simulink model "CMOS_Kernel_Memory_Sync"  (R2023b)
settings: Solver=VariableStepAuto  StartTime=0.0  StopTime=30000000  RelTol=1e-3
values from neighbouring files (symbols this model uses):
  AmountOfPixelsPerScanline = 400    [Kernel_Setup_Script.m]
  AmountOfRamBlocksScanlines = 5    [Kernel_Setup_Script.m]
  AmountOfRamBlocksScanlinesOffset = AmountOfRamBlocksScanlines - 1    (= 4)    [Kernel_Setup_Script.m]
  AmountOfScanlinePixels = 73700    [Kernel_Setup_Script.m]
  AmountOfScanlinePixelsOffset = AmountOfScanlinePixels - 1    (= 73699)    [Kernel_Setup_Script.m]
  AmountOfScanlines = 1100    [Kernel_Setup_Script.m]
  AmountOfScanlinesOffset = AmountOfScanlines - 1    (= 1099)    [Kernel_Setup_Script.m]
  AOPPK_Off = AmountOfPixelsPerScanline - 1    (= 399)    [Kernel_Setup_Script.m]
  AOPPS_Off = AmountOfPixelsPerScanline - 1    (= 399)    [Kernel_Setup_Script.m]
  FramePackOff_0 = FramePackOff_0 - ScanlineFifoCheck    [Kernel_Setup_Script.m]
  FramePackOff_1 = FramePackOff_1 - ScanlineFifoCheck    [Kernel_Setup_Script.m]
  FramePackOff_2 = FramePackOff_2 - ScanlineFifoCheck    [Kernel_Setup_Script.m]
  FramePackOff_3 = FramePackOff_3 - ScanlineFifoCheck    [Kernel_Setup_Script.m]
  FramePackOff_4 = FramePackOff_4 - ScanlineFifoCheck    [Kernel_Setup_Script.m]
  FramePackOff_5 = FramePackOff_5 - ScanlineFifoCheck    [Kernel_Setup_Script.m]
  KernelPackOff_0 = KernelPackOff_0 - KernelBitsPerRow    [Kernel_Setup_Script.m]
  KernelPackOff_1 = KernelPackOff_1 - KernelBitsPerRow    [Kernel_Setup_Script.m]
  KernelPackOff_2 = KernelPackOff_2 - KernelBitsPerRow    [Kernel_Setup_Script.m]
  KernelPackOff_3 = KernelPackOff_3 - KernelBitsPerRow    [Kernel_Setup_Script.m]
  Slice59DownTo48Top = (MsbOffset - (ScanlinePixelBitSizeController*1))    (= 59)    [Kernel_Setup_Script.m]
  Slice71DownTo60Top = (MsbOffset - (ScanlinePixelBitSizeController*0))    (= 71)    [Kernel_Setup_Script.m]
  TotalSectionsForFrames = AmountOfScanlines/AmountOfRamBlocksScanlines    (= 220)    [Kernel_Setup_Script.m]
  UltraRamRows = AmountOfPixelsPerScanline/ScanlineFifoCheck    [Kernel_Setup_Script.m]
  UltraRamRowsCeil = ceil(AmountOfPixelsPerScanline/ScanlineFifoCheck)    [Kernel_Setup_Script.m]
  UltraRamRowsKernel = AmountOfPixelsPerScanline/KernelBitsPerRow    (= 100)    [Kernel_Setup_Script.m]
  UltraRamRowsKernelCeil = ceil(AmountOfPixelsPerScanline/KernelBitsPerRow)    [Kernel_Setup_Script.m]
  UltraRamRowsMemorySectionOffset = UltraRamRowsCeil*AmountOfRamBlocksScanlines    [Kernel_Setup_Script.m]
  UltraRamRowsOffset = UltraRamRowsCeil - 1    [Kernel_Setup_Script.m]
undefined symbols (not defined in the file or in its folder): c, Down, sfvc784, Up, xck26
libraries: hdlBasic x4512, vmcUtilities x1
(part 4 of 39)

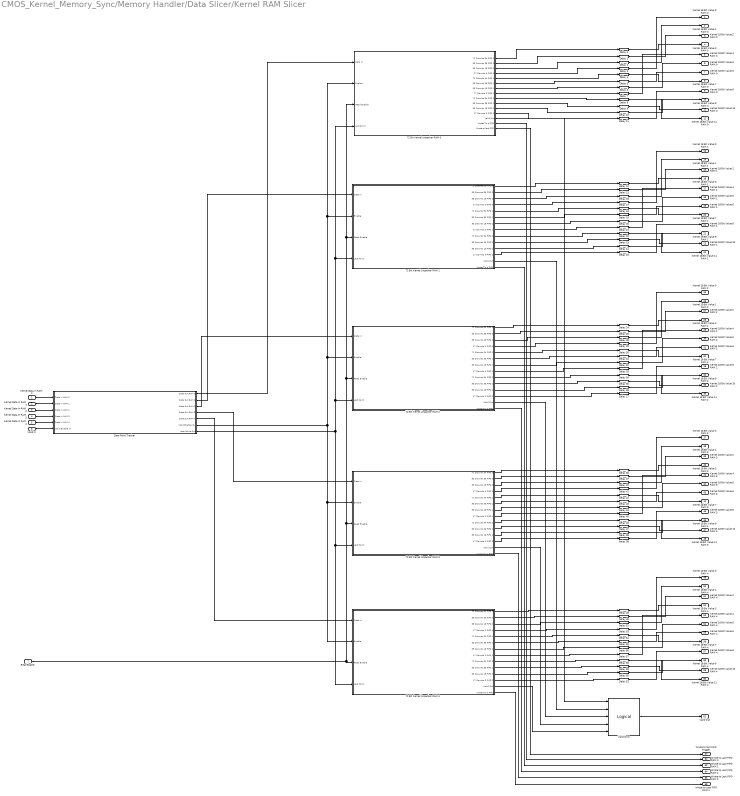
== system CMOS_Kernel_Memory_Sync/Memory Handler/Data Slicer/Kernel RAM Slicer ==
  Kernel Data In RAM 0 : Inport
  Kernel Data In RAM 1 : Inport  Port=2
  Kernel Data In RAM 2 : Inport  Port=3
  Kernel Data In RAM 3 : Inport  Port=4
  Kernel Data In RAM 4 : Inport  Port=5
  Valid In : Inport  Port=6
  Read Enable : Inport  Port=7
  72 Bit Kernel Unpacker RAM 0 : Subsystem
      settings: RTWMemSecFuncInitTerm=Inherit fRAM model  RTWMemSecFuncExecute=Inherit fRAM model  RTWMemSecDataConstants=Inherit fRAM model  RTWMemSecDataInternal=Inherit fRAM model  RTWMemSecDataParameters=Inherit fRAM model
  72 Bit Kernel Unpacker RAM 1 : Subsystem
      settings: RTWMemSecFuncInitTerm=Inherit fRAM model  RTWMemSecFuncExecute=Inherit fRAM model  RTWMemSecDataConstants=Inherit fRAM model  RTWMemSecDataInternal=Inherit fRAM model  RTWMemSecDataParameters=Inherit fRAM model
  72 Bit Kernel Unpacker RAM 2 : Subsystem
      settings: RTWMemSecFuncInitTerm=Inherit fRAM model  RTWMemSecFuncExecute=Inherit fRAM model  RTWMemSecDataConstants=Inherit fRAM model  RTWMemSecDataInternal=Inherit fRAM model  RTWMemSecDataParameters=Inherit fRAM model
  72 Bit Kernel Unpacker RAM 3 : Subsystem
      settings: RTWMemSecFuncInitTerm=Inherit fRAM model  RTWMemSecFuncExecute=Inherit fRAM model  RTWMemSecDataConstants=Inherit fRAM model  RTWMemSecDataInternal=Inherit fRAM model  RTWMemSecDataParameters=Inherit fRAM model
  72 Bit Kernel Unpacker RAM 4 : Subsystem
      settings: RTWMemSecFuncInitTerm=Inherit fRAM model  RTWMemSecFuncExecute=Inherit fRAM model  RTWMemSecDataConstants=Inherit fRAM model  RTWMemSecDataInternal=Inherit fRAM model  RTWMemSecDataParameters=Inherit fRAM model
  Data Point Tracker : Subsystem
  Delay {0..59} (60 alike) : hdlBasic/Delay  rst=off  en=off  latency=1  reg_retiming=off  XmcBlockStatus=1  maskContainerNames=group1  block_type=delay  block_config=sysgen:Delay_config
  Valid Sync : hdlBasic/Logical  logical_function=AND  inputs=5  en=off  latency=1  precision=Full  arith_type=Unsigned  n_bits=16  bin_pt=0  align_bp=on  overflow=[]  quantization=[]  XmcBlockStatus=1  maskContainerNames=tabcontainer1  block_type=logical  block_config=sysgen:Logical_config
  Kernel 18 Bit Value 0 RAM 0 : Outport
  Kernel 18 Bit Value 1 RAM 0 : Outport  Port=2
  Kernel 18 Bit Value 2 RAM 0 : Outport  Port=3
  Kernel 18 Bit Value 3 RAM 0 : Outport  Port=4
  Kernel 18 Bit Value 4 RAM 0 : Outport  Port=5
  Kernel 18 Bit Value 5 RAM 0 : Outport  Port=6
  Kernel 18 Bit Value 6 RAM 0 : Outport  Port=7
  Kernel 18 Bit Value 7 RAM 0 : Outport  Port=8
  Kernel 18 Bit Value 8 RAM 0 : Outport  Port=9
  Kernel 18 Bit Value 9 RAM 0 : Outport  Port=10
  Kernel 18 Bit Value 10 RAM 0 : Outport  Port=11
  Kernel 18 Bit Value 11 RAM 0 : Outport  Port=12
  Kernel 18 Bit Value 0 RAM 1 : Outport  Port=13
  Kernel 18 Bit Value 1 RAM 1 : Outport  Port=14
  Kernel 18 Bit Value 2 RAM 1 : Outport  Port=15
  Kernel 18 Bit Value 3 RAM 1 : Outport  Port=16
  Kernel 18 Bit Value 4 RAM 1 : Outport  Port=17
  Kernel 18 Bit Value 5 RAM 1 : Outport  Port=18
  Kernel 18 Bit Value 6 RAM 1 : Outport  Port=19
  Kernel 18 Bit Value 7 RAM 1 : Outport  Port=20
  Kernel 18 Bit Value 8 RAM 1 : Outport  Port=21
  Kernel 18 Bit Value 9 RAM 1 : Outport  Port=22
  Kernel 18 Bit Value 10 RAM 1 : Outport  Port=23
  Kernel 18 Bit Value 11 RAM 1 : Outport  Port=24
  Kernel 18 Bit Value 0 RAM 2 : Outport  Port=25
  Kernel 18 Bit Value 1 RAM 2 : Outport  Port=26
  Kernel 18 Bit Value 2 RAM 2 : Outport  Port=27
  Kernel 18 Bit Value 3 RAM 2 : Outport  Port=28
  Kernel 18 Bit Value 4 RAM 2 : Outport  Port=29
  Kernel 18 Bit Value 5 RAM 2 : Outport  Port=30
  Kernel 18 Bit Value 6 RAM 2 : Outport  Port=31
  Kernel 18 Bit Value 7 RAM 2 : Outport  Port=32
  Kernel 18 Bit Value 8 RAM 2 : Outport  Port=33
  Kernel 18 Bit Value 9 RAM 2 : Outport  Port=34
  Kernel 18 Bit Value 10 RAM 2 : Outport  Port=35
  Kernel 18 Bit Value 11 RAM 2 : Outport  Port=36
  Kernel 18 Bit Value 0 RAM 3 : Outport  Port=37
  Kernel 18 Bit Value 1 RAM 3 : Outport  Port=38
  Kernel 18 Bit Value 2 RAM 3 : Outport  Port=39
  Kernel 18 Bit Value 3 RAM 3 : Outport  Port=40
  Kernel 18 Bit Value 4 RAM 3 : Outport  Port=41
  Kernel 18 Bit Value 5 RAM 3 : Outport  Port=42
  Kernel 18 Bit Value 6 RAM 3 : Outport  Port=43
  Kernel 18 Bit Value 7 RAM 3 : Outport  Port=44
  Kernel 18 Bit Value 8 RAM 3 : Outport  Port=45
  Kernel 18 Bit Value 9 RAM 3 : Outport  Port=46
  Kernel 18 Bit Value 10 RAM 3 : Outport  Port=47
  Kernel 18 Bit Value 11 RAM 3 : Outport  Port=48
  Kernel 18 Bit Value 0 RAM 4 : Outport  Port=49
  Kernel 18 Bit Value 1 RAM 4 : Outport  Port=50
  Kernel 18 Bit Value 2 RAM 4 : Outport  Port=51
  Kernel 18 Bit Value 3 RAM 4 : Outport  Port=52
  Kernel 18 Bit Value 4 RAM 4 : Outport  Port=53
  Kernel 18 Bit Value 5 RAM 4 : Outport  Port=54
  Kernel 18 Bit Value 6 RAM 4 : Outport  Port=55
  Kernel 18 Bit Value 7 RAM 4 : Outport  Port=56
  Kernel 18 Bit Value 8 RAM 4 : Outport  Port=57
  Kernel 18 Bit Value 9 RAM 4 : Outport  Port=58
  Kernel 18 Bit Value 10 RAM 4 : Outport  Port=59
  Kernel 18 Bit Value 11 RAM 4 : Outport  Port=60
  Valid Out : Outport  Port=61
  Wrote to Last FIFO RAM 0 : Outport  Port=62
  Wrote to Last FIFO RAM 1 : Outport  Port=63
  Wrote to Last FIFO RAM 2 : Outport  Port=64
  Wrote to Last FIFO RAM 3 : Outport  Port=65
  Wrote to Last FIFO RAM 4 : Outport  Port=66
  Wrote to last FIFO Trigger : Outport  Port=67
  wires:
  72 Bit Kernel Unpacker RAM 0/4(17 Downto 0 FIFO 0) -> Delay 3/1
  72 Bit Kernel Unpacker RAM 0/3(35 Downto 18 FIFO 0) -> Delay 2/1
  72 Bit Kernel Unpacker RAM 0/2(53 Downto 36 FIFO 0) -> Delay 1/1
  72 Bit Kernel Unpacker RAM 0/1(71 Downto 54 FIFO 0) -> Delay 0/1
  72 Bit Kernel Unpacker RAM 0/8(17 Downto 0 FIFO 1) -> Delay 7/1
  72 Bit Kernel Unpacker RAM 0/7(35 Downto 18 FIFO 1) -> Delay 6/1
  72 Bit Kernel Unpacker RAM 0/6(53 Downto 36 FIFO 1) -> Delay 5/1
  72 Bit Kernel Unpacker RAM 0/5(71 Downto 54 FIFO 1) -> Delay 4/1
  72 Bit Kernel Unpacker RAM 0/12(17 Downto 0 FIFO 2) -> Delay 11/1
  72 Bit Kernel Unpacker RAM 0/11(35 Downto 18 FIFO 2) -> Delay 10/1
  72 Bit Kernel Unpacker RAM 0/10(53 Downto 36 FIFO 2) -> Delay 9/1
  72 Bit Kernel Unpacker RAM 0/9(71 Downto 54 FIFO 2) -> Delay 8/1
  Delay 0/1 -> Kernel 18 Bit Value 3 RAM 0/1
  Delay 1/1 -> Kernel 18 Bit Value 2 RAM 0/1
  Delay 2/1 -> Kernel 18 Bit Value 1 RAM 0/1
  Delay 3/1 -> Kernel 18 Bit Value 0 RAM 0/1
  Delay 4/1 -> Kernel 18 Bit Value 7 RAM 0/1
  Delay 5/1 -> Kernel 18 Bit Value 6 RAM 0/1
  Delay 6/1 -> Kernel 18 Bit Value 5 RAM 0/1
  Delay 7/1 -> Kernel 18 Bit Value 4 RAM 0/1
  Delay 8/1 -> Kernel 18 Bit Value 11 RAM 0/1
  Delay 9/1 -> Kernel 18 Bit Value 10 RAM 0/1
  Delay 10/1 -> Kernel 18 Bit Value 9 RAM 0/1
  Delay 11/1 -> Kernel 18 Bit Value 8 RAM 0/1
  Delay 18/1 -> Kernel 18 Bit Value 7 RAM 1/1
  Delay 17/1 -> Kernel 18 Bit Value 0 RAM 1/1
  Delay 12/1 -> Kernel 18 Bit Value 3 RAM 1/1
  72 Bit Kernel Unpacker RAM 1/3(35 Downto 18 FIFO 0) -> Delay 16/1
  72 Bit Kernel Unpacker RAM 1/9(71 Downto 54 FIFO 2) -> Delay 22/1
  Delay 21/1 -> Kernel 18 Bit Value 4 RAM 1/1
  Delay 19/1 -> Kernel 18 Bit Value 6 RAM 1/1
  Delay 20/1 -> Kernel 18 Bit Value 5 RAM 1/1
  72 Bit Kernel Unpacker RAM 1/8(17 Downto 0 FIFO 1) -> Delay 21/1
  Delay 16/1 -> Kernel 18 Bit Value 1 RAM 1/1
  72 Bit Kernel Unpacker RAM 1/7(35 Downto 18 FIFO 1) -> Delay 20/1
  72 Bit Kernel Unpacker RAM 1/1(71 Downto 54 FIFO 0) -> Delay 12/1
  Delay 23/1 -> Kernel 18 Bit Value 10 RAM 1/1
  72 Bit Kernel Unpacker RAM 1/10(53 Downto 36 FIFO 2) -> Delay 23/1
  Delay 22/1 -> Kernel 18 Bit Value 11 RAM 1/1
  Delay 13/1 -> Kernel 18 Bit Value 2 RAM 1/1
  72 Bit Kernel Unpacker RAM 1/2(53 Downto 36 FIFO 0) -> Delay 13/1
  72 Bit Kernel Unpacker RAM 1/4(17 Downto 0 FIFO 0) -> Delay 17/1
  72 Bit Kernel Unpacker RAM 1/12(17 Downto 0 FIFO 2) -> Delay 15/1
  72 Bit Kernel Unpacker RAM 1/11(35 Downto 18 FIFO 2) -> Delay 14/1
  Delay 14/1 -> Kernel 18 Bit Value 9 RAM 1/1
  72 Bit Kernel Unpacker RAM 1/6(53 Downto 36 FIFO 1) -> Delay 19/1
  Delay 15/1 -> Kernel 18 Bit Value 8 RAM 1/1
  72 Bit Kernel Unpacker RAM 1/5(71 Downto 54 FIFO 1) -> Delay 18/1
  Delay 30/1 -> Kernel 18 Bit Value 7 RAM 2/1
  Delay 29/1 -> Kernel 18 Bit Value 0 RAM 2/1
  Delay 24/1 -> Kernel 18 Bit Value 3 RAM 2/1
  72 Bit Kernel Unpacker RAM 2/3(35 Downto 18 FIFO 0) -> Delay 28/1
  72 Bit Kernel Unpacker RAM 2/9(71 Downto 54 FIFO 2) -> Delay 34/1
  Delay 33/1 -> Kernel 18 Bit Value 4 RAM 2/1
  Delay 31/1 -> Kernel 18 Bit Value 6 RAM 2/1
  Delay 32/1 -> Kernel 18 Bit Value 5 RAM 2/1
  72 Bit Kernel Unpacker RAM 2/8(17 Downto 0 FIFO 1) -> Delay 33/1
  Delay 28/1 -> Kernel 18 Bit Value 1 RAM 2/1
  72 Bit Kernel Unpacker RAM 2/7(35 Downto 18 FIFO 1) -> Delay 32/1
  72 Bit Kernel Unpacker RAM 2/1(71 Downto 54 FIFO 0) -> Delay 24/1
  Delay 35/1 -> Kernel 18 Bit Value 10 RAM 2/1
  72 Bit Kernel Unpacker RAM 2/10(53 Downto 36 FIFO 2) -> Delay 35/1
  Delay 34/1 -> Kernel 18 Bit Value 11 RAM 2/1
  Delay 25/1 -> Kernel 18 Bit Value 2 RAM 2/1
  72 Bit Kernel Unpacker RAM 2/2(53 Downto 36 FIFO 0) -> Delay 25/1
  72 Bit Kernel Unpacker RAM 2/4(17 Downto 0 FIFO 0) -> Delay 29/1
  72 Bit Kernel Unpacker RAM 2/12(17 Downto 0 FIFO 2) -> Delay 27/1
  72 Bit Kernel Unpacker RAM 2/11(35 Downto 18 FIFO 2) -> Delay 26/1
  Delay 26/1 -> Kernel 18 Bit Value 9 RAM 2/1
  72 Bit Kernel Unpacker RAM 2/6(53 Downto 36 FIFO 1) -> Delay 31/1
  Delay 27/1 -> Kernel 18 Bit Value 8 RAM 2/1
  72 Bit Kernel Unpacker RAM 2/5(71 Downto 54 FIFO 1) -> Delay 30/1
  Delay 42/1 -> Kernel 18 Bit Value 7 RAM 3/1
  Delay 41/1 -> Kernel 18 Bit Value 0 RAM 3/1
  Delay 36/1 -> Kernel 18 Bit Value 3 RAM 3/1
  72 Bit Kernel Unpacker RAM 3/3(35 Downto 18 FIFO 0) -> Delay 40/1
  72 Bit Kernel Unpacker RAM 3/9(71 Downto 54 FIFO 2) -> Delay 46/1
  Delay 45/1 -> Kernel 18 Bit Value 4 RAM 3/1
  Delay 43/1 -> Kernel 18 Bit Value 6 RAM 3/1
  Delay 44/1 -> Kernel 18 Bit Value 5 RAM 3/1
  72 Bit Kernel Unpacker RAM 3/8(17 Downto 0 FIFO 1) -> Delay 45/1
  Delay 40/1 -> Kernel 18 Bit Value 1 RAM 3/1
  72 Bit Kernel Unpacker RAM 3/7(35 Downto 18 FIFO 1) -> Delay 44/1
  72 Bit Kernel Unpacker RAM 3/1(71 Downto 54 FIFO 0) -> Delay 36/1
  Delay 47/1 -> Kernel 18 Bit Value 10 RAM 3/1
  72 Bit Kernel Unpacker RAM 3/10(53 Downto 36 FIFO 2) -> Delay 47/1
  Delay 46/1 -> Kernel 18 Bit Value 11 RAM 3/1
  Delay 37/1 -> Kernel 18 Bit Value 2 RAM 3/1
  72 Bit Kernel Unpacker RAM 3/2(53 Downto 36 FIFO 0) -> Delay 37/1
  72 Bit Kernel Unpacker RAM 3/4(17 Downto 0 FIFO 0) -> Delay 41/1
  72 Bit Kernel Unpacker RAM 3/12(17 Downto 0 FIFO 2) -> Delay 39/1
  72 Bit Kernel Unpacker RAM 3/11(35 Downto 18 FIFO 2) -> Delay 38/1
  Delay 38/1 -> Kernel 18 Bit Value 9 RAM 3/1
  72 Bit Kernel Unpacker RAM 3/6(53 Downto 36 FIFO 1) -> Delay 43/1
  Delay 39/1 -> Kernel 18 Bit Value 8 RAM 3/1
  72 Bit Kernel Unpacker RAM 3/5(71 Downto 54 FIFO 1) -> Delay 42/1
  Delay 54/1 -> Kernel 18 Bit Value 7 RAM 4/1
  Delay 53/1 -> Kernel 18 Bit Value 0 RAM 4/1
  Delay 48/1 -> Kernel 18 Bit Value 3 RAM 4/1
  72 Bit Kernel Unpacker RAM 4/3(35 Downto 18 FIFO 0) -> Delay 52/1
  72 Bit Kernel Unpacker RAM 4/9(71 Downto 54 FIFO 2) -> Delay 58/1
  Delay 57/1 -> Kernel 18 Bit Value 4 RAM 4/1
  Delay 55/1 -> Kernel 18 Bit Value 6 RAM 4/1
  Delay 56/1 -> Kernel 18 Bit Value 5 RAM 4/1
  72 Bit Kernel Unpacker RAM 4/8(17 Downto 0 FIFO 1) -> Delay 57/1
  Delay 52/1 -> Kernel 18 Bit Value 1 RAM 4/1
  72 Bit Kernel Unpacker RAM 4/7(35 Downto 18 FIFO 1) -> Delay 56/1
  72 Bit Kernel Unpacker RAM 4/1(71 Downto 54 FIFO 0) -> Delay 48/1
  Delay 59/1 -> Kernel 18 Bit Value 10 RAM 4/1
  72 Bit Kernel Unpacker RAM 4/10(53 Downto 36 FIFO 2) -> Delay 59/1
  Delay 58/1 -> Kernel 18 Bit Value 11 RAM 4/1
  Delay 49/1 -> Kernel 18 Bit Value 2 RAM 4/1
  72 Bit Kernel Unpacker RAM 4/2(53 Downto 36 FIFO 0) -> Delay 49/1
  72 Bit Kernel Unpacker RAM 4/4(17 Downto 0 FIFO 0) -> Delay 53/1
  72 Bit Kernel Unpacker RAM 4/12(17 Downto 0 FIFO 2) -> Delay 51/1
  72 Bit Kernel Unpacker RAM 4/11(35 Downto 18 FIFO 2) -> Delay 50/1
  Delay 50/1 -> Kernel 18 Bit Value 9 RAM 4/1
  72 Bit Kernel Unpacker RAM 4/6(53 Downto 36 FIFO 1) -> Delay 55/1
  Delay 51/1 -> Kernel 18 Bit Value 8 RAM 4/1
  72 Bit Kernel Unpacker RAM 4/5(71 Downto 54 FIFO 1) -> Delay 54/1
  Valid Sync/1 -> Valid Out/1
  72 Bit Kernel Unpacker RAM 0/13(Valid Out) -> Valid Sync/1
  72 Bit Kernel Unpacker RAM 1/13(Valid Out) -> Valid Sync/2
  72 Bit Kernel Unpacker RAM 2/13(Valid Out) -> Valid Sync/3
  72 Bit Kernel Unpacker RAM 3/13(Valid Out) -> Valid Sync/4
  72 Bit Kernel Unpacker RAM 4/13(Valid Out) -> Valid Sync/5
  Read Enable/1 -> 72 Bit Kernel Unpacker RAM 4/3(Read Enable), 72 Bit Kernel Unpacker RAM 3/3(Read Enable), 72 Bit Kernel Unpacker RAM 2/3(Read Enable), 72 Bit Kernel Unpacker RAM 1/3(Read Enable), 72 Bit Kernel Unpacker RAM 0/3(Read Enable)
  Kernel Data In RAM 0/1 -> Data Point Tracker/1(Data In RAM 0)
  Data Point Tracker/1(Data Out RAM 0) -> 72 Bit Kernel Unpacker RAM 0/1(Data In)
  Kernel Data In RAM 1/1 -> Data Point Tracker/2(Data In RAM 1)
  Data Point Tracker/2(Data Out RAM 1) -> 72 Bit Kernel Unpacker RAM 1/1(Data In)
  Kernel Data In RAM 2/1 -> Data Point Tracker/3(Data In RAM 2)
  Data Point Tracker/3(Data Out RAM 2) -> 72 Bit Kernel Unpacker RAM 2/1(Data In)
  Kernel Data In RAM 3/1 -> Data Point Tracker/4(Data In RAM 3)
  Data Point Tracker/4(Data Out RAM 3) -> 72 Bit Kernel Unpacker RAM 3/1(Data In)
  Kernel Data In RAM 4/1 -> Data Point Tracker/5(Data In RAM 4)
  Valid In/1 -> Data Point Tracker/6(Valid Enable In)
  Data Point Tracker/5(Data Out RAM 4) -> 72 Bit Kernel Unpacker RAM 4/1(Data In)
  Data Point Tracker/6(Valid Enable Out) -> 72 Bit Kernel Unpacker RAM 4/2(Enable), 72 Bit Kernel Unpacker RAM 3/2(Enable), 72 Bit Kernel Unpacker RAM 2/2(Enable), 72 Bit Kernel Unpacker RAM 1/2(Enable), 72 Bit Kernel Unpacker RAM 0/2(Enable)
  Data Point Tracker/7(Last Value Out) -> 72 Bit Kernel Unpacker RAM 4/4(Last Point), 72 Bit Kernel Unpacker RAM 3/4(Last Point), 72 Bit Kernel Unpacker RAM 2/4(Last Point), 72 Bit Kernel Unpacker RAM 1/4(Last Point), 72 Bit Kernel Unpacker RAM 0/4(Last Point)
  72 Bit Kernel Unpacker RAM 0/14(Wrote To a FIFO) -> Wrote to Last FIFO RAM 0/1
  72 Bit Kernel Unpacker RAM 1/14(Wrote To a FIFO) -> Wrote to Last FIFO RAM 1/1
  72 Bit Kernel Unpacker RAM 2/14(Wrote To a FIFO) -> Wrote to Last FIFO RAM 2/1
  72 Bit Kernel Unpacker RAM 3/14(Wrote To a FIFO) -> Wrote to Last FIFO RAM 3/1
  72 Bit Kernel Unpacker RAM 4/14(Wrote To a FIFO) -> Wrote to Last FIFO RAM 4/1
  72 Bit Kernel Unpacker RAM 0/15(Wrote to last FIFO) -> Wrote to last FIFO Trigger/1

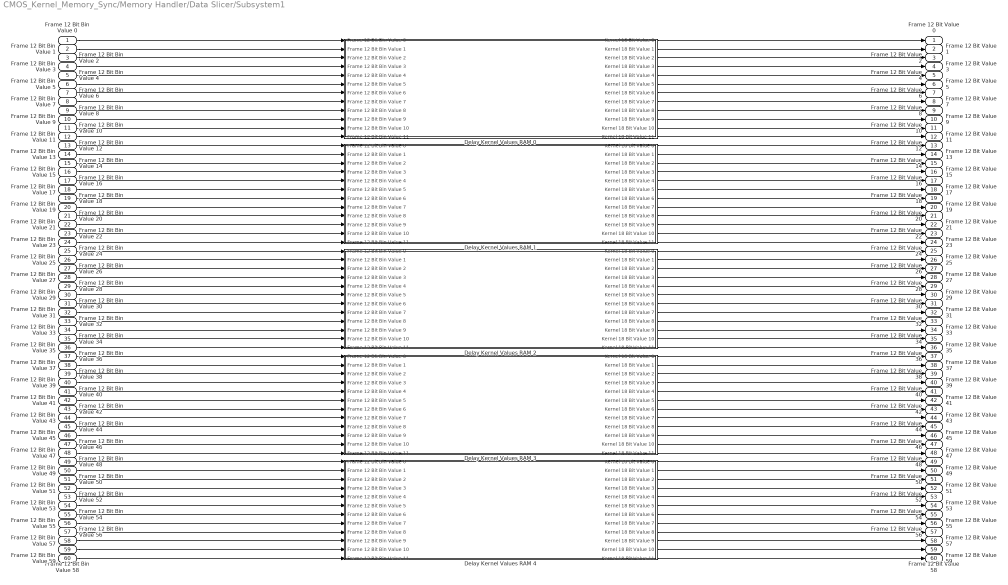
== system CMOS_Kernel_Memory_Sync/Memory Handler/Data Slicer/Subsystem1 ==
  Frame 12 Bit Bin Value 0 : Inport
  Frame 12 Bit Bin Value 1 : Inport  Port=2
  Frame 12 Bit Bin Value 2 : Inport  Port=3
  Frame 12 Bit Bin Value 3 : Inport  Port=4
  Frame 12 Bit Bin Value 4 : Inport  Port=5
  Frame 12 Bit Bin Value 5 : Inport  Port=6
  Frame 12 Bit Bin Value 6 : Inport  Port=7
  Frame 12 Bit Bin Value 7 : Inport  Port=8
  Frame 12 Bit Bin Value 8 : Inport  Port=9
  Frame 12 Bit Bin Value 9 : Inport  Port=10
  Frame 12 Bit Bin Value 10 : Inport  Port=11
  Frame 12 Bit Bin Value 11 : Inport  Port=12
  Frame 12 Bit Bin Value 12 : Inport  Port=13
  Frame 12 Bit Bin Value 13 : Inport  Port=14
  Frame 12 Bit Bin Value 14 : Inport  Port=15
  Frame 12 Bit Bin Value 15 : Inport  Port=16
  Frame 12 Bit Bin Value 16 : Inport  Port=17
  Frame 12 Bit Bin Value 17 : Inport  Port=18
  Frame 12 Bit Bin Value 18 : Inport  Port=19
  Frame 12 Bit Bin Value 19 : Inport  Port=20
  Frame 12 Bit Bin Value 20 : Inport  Port=21
  Frame 12 Bit Bin Value 21 : Inport  Port=22
  Frame 12 Bit Bin Value 22 : Inport  Port=23
  Frame 12 Bit Bin Value 23 : Inport  Port=24
  Frame 12 Bit Bin Value 24 : Inport  Port=25
  Frame 12 Bit Bin Value 25 : Inport  Port=26
  Frame 12 Bit Bin Value 26 : Inport  Port=27
  Frame 12 Bit Bin Value 27 : Inport  Port=28
  Frame 12 Bit Bin Value 28 : Inport  Port=29
  Frame 12 Bit Bin Value 29 : Inport  Port=30
  Frame 12 Bit Bin Value 30 : Inport  Port=31
  Frame 12 Bit Bin Value 31 : Inport  Port=32
  Frame 12 Bit Bin Value 32 : Inport  Port=33
  Frame 12 Bit Bin Value 33 : Inport  Port=34
  Frame 12 Bit Bin Value 34 : Inport  Port=35
  Frame 12 Bit Bin Value 35 : Inport  Port=36
  Frame 12 Bit Bin Value 36 : Inport  Port=37
  Frame 12 Bit Bin Value 37 : Inport  Port=38
  Frame 12 Bit Bin Value 38 : Inport  Port=39
  Frame 12 Bit Bin Value 39 : Inport  Port=40
  Frame 12 Bit Bin Value 40 : Inport  Port=41
  Frame 12 Bit Bin Value 41 : Inport  Port=42
  Frame 12 Bit Bin Value 42 : Inport  Port=43
  Frame 12 Bit Bin Value 43 : Inport  Port=44
  Frame 12 Bit Bin Value 44 : Inport  Port=45
  Frame 12 Bit Bin Value 45 : Inport  Port=46
  Frame 12 Bit Bin Value 46 : Inport  Port=47
  Frame 12 Bit Bin Value 47 : Inport  Port=48
  Frame 12 Bit Bin Value 48 : Inport  Port=49
  Frame 12 Bit Bin Value 49 : Inport  Port=50
  Frame 12 Bit Bin Value 50 : Inport  Port=51
  Frame 12 Bit Bin Value 51 : Inport  Port=52
  Frame 12 Bit Bin Value 52 : Inport  Port=53
  Frame 12 Bit Bin Value 53 : Inport  Port=54
  Frame 12 Bit Bin Value 54 : Inport  Port=55
  Frame 12 Bit Bin Value 55 : Inport  Port=56
  Frame 12 Bit Bin Value 56 : Inport  Port=57
  Frame 12 Bit Bin Value 57 : Inport  Port=58
  Frame 12 Bit Bin Value 58 : Inport  Port=59
  Frame 12 Bit Bin Value 59 : Inport  Port=60
  Delay Kernel Values RAM 0 : Subsystem
      settings: RTWMemSecFuncInitTerm=Inherit fRAM model  RTWMemSecFuncExecute=Inherit fRAM model  RTWMemSecDataConstants=Inherit fRAM model  RTWMemSecDataInternal=Inherit fRAM model  RTWMemSecDataParameters=Inherit fRAM model
  Delay Kernel Values RAM 1 : Subsystem
      settings: RTWMemSecFuncInitTerm=Inherit fRAM model  RTWMemSecFuncExecute=Inherit fRAM model  RTWMemSecDataConstants=Inherit fRAM model  RTWMemSecDataInternal=Inherit fRAM model  RTWMemSecDataParameters=Inherit fRAM model
  Delay Kernel Values RAM 2 : Subsystem
      settings: RTWMemSecFuncInitTerm=Inherit fRAM model  RTWMemSecFuncExecute=Inherit fRAM model  RTWMemSecDataConstants=Inherit fRAM model  RTWMemSecDataInternal=Inherit fRAM model  RTWMemSecDataParameters=Inherit fRAM model
  Delay Kernel Values RAM 3 : Subsystem
      settings: RTWMemSecFuncInitTerm=Inherit fRAM model  RTWMemSecFuncExecute=Inherit fRAM model  RTWMemSecDataConstants=Inherit fRAM model  RTWMemSecDataInternal=Inherit fRAM model  RTWMemSecDataParameters=Inherit fRAM model
  Delay Kernel Values RAM 4 : Subsystem
      settings: RTWMemSecFuncInitTerm=Inherit fRAM model  RTWMemSecFuncExecute=Inherit fRAM model  RTWMemSecDataConstants=Inherit fRAM model  RTWMemSecDataInternal=Inherit fRAM model  RTWMemSecDataParameters=Inherit fRAM model
  Frame 12 Bit Value 0 : Outport
  Frame 12 Bit Value 1 : Outport  Port=2
  Frame 12 Bit Value 2 : Outport  Port=3
  Frame 12 Bit Value 3 : Outport  Port=4
  Frame 12 Bit Value 4 : Outport  Port=5
  Frame 12 Bit Value 5 : Outport  Port=6
  Frame 12 Bit Value 6 : Outport  Port=7
  Frame 12 Bit Value 7 : Outport  Port=8
  Frame 12 Bit Value 8 : Outport  Port=9
  Frame 12 Bit Value 9 : Outport  Port=10
  Frame 12 Bit Value 10 : Outport  Port=11
  Frame 12 Bit Value 11 : Outport  Port=12
  Frame 12 Bit Value 12 : Outport  Port=13
  Frame 12 Bit Value 13 : Outport  Port=14
  Frame 12 Bit Value 14 : Outport  Port=15
  Frame 12 Bit Value 15 : Outport  Port=16
  Frame 12 Bit Value 16 : Outport  Port=17
  Frame 12 Bit Value 17 : Outport  Port=18
  Frame 12 Bit Value 18 : Outport  Port=19
  Frame 12 Bit Value 19 : Outport  Port=20
  Frame 12 Bit Value 20 : Outport  Port=21
  Frame 12 Bit Value 21 : Outport  Port=22
  Frame 12 Bit Value 22 : Outport  Port=23
  Frame 12 Bit Value 23 : Outport  Port=24
  Frame 12 Bit Value 24 : Outport  Port=25
  Frame 12 Bit Value 25 : Outport  Port=26
  Frame 12 Bit Value 26 : Outport  Port=27
  Frame 12 Bit Value 27 : Outport  Port=28
  Frame 12 Bit Value 28 : Outport  Port=29
  Frame 12 Bit Value 29 : Outport  Port=30
  Frame 12 Bit Value 30 : Outport  Port=31
  Frame 12 Bit Value 31 : Outport  Port=32
  Frame 12 Bit Value 32 : Outport  Port=33
  Frame 12 Bit Value 33 : Outport  Port=34
  Frame 12 Bit Value 34 : Outport  Port=35
  Frame 12 Bit Value 35 : Outport  Port=36
  Frame 12 Bit Value 36 : Outport  Port=37
  Frame 12 Bit Value 37 : Outport  Port=38
  Frame 12 Bit Value 38 : Outport  Port=39
  Frame 12 Bit Value 39 : Outport  Port=40
  Frame 12 Bit Value 40 : Outport  Port=41
  Frame 12 Bit Value 41 : Outport  Port=42
  Frame 12 Bit Value 42 : Outport  Port=43
  Frame 12 Bit Value 43 : Outport  Port=44
  Frame 12 Bit Value 44 : Outport  Port=45
  Frame 12 Bit Value 45 : Outport  Port=46
  Frame 12 Bit Value 46 : Outport  Port=47
  Frame 12 Bit Value 47 : Outport  Port=48
  Frame 12 Bit Value 48 : Outport  Port=49
  Frame 12 Bit Value 49 : Outport  Port=50
  Frame 12 Bit Value 50 : Outport  Port=51
  Frame 12 Bit Value 51 : Outport  Port=52
  Frame 12 Bit Value 52 : Outport  Port=53
  Frame 12 Bit Value 53 : Outport  Port=54
  Frame 12 Bit Value 54 : Outport  Port=55
  Frame 12 Bit Value 55 : Outport  Port=56
  Frame 12 Bit Value 56 : Outport  Port=57
  Frame 12 Bit Value 57 : Outport  Port=58
  Frame 12 Bit Value 58 : Outport  Port=59
  Frame 12 Bit Value 59 : Outport  Port=60
  wires:
  Delay Kernel Values RAM 2/4(Kernel 18 Bit Value 3) -> Frame 12 Bit Value 27/1
  Frame 12 Bit Bin Value 2/1 -> Delay Kernel Values RAM 0/3(Frame 12 Bit Bin Value 2)
  Frame 12 Bit Bin Value 26/1 -> Delay Kernel Values RAM 2/3(Frame 12 Bit Bin Value 2)
  Frame 12 Bit Bin Value 21/1 -> Delay Kernel Values RAM 1/10(Frame 12 Bit Bin Value 9)
  Frame 12 Bit Bin Value 37/1 -> Delay Kernel Values RAM 3/2(Frame 12 Bit Bin Value 1)
  Delay Kernel Values RAM 0/7(Kernel 18 Bit Value 6) -> Frame 12 Bit Value 6/1
  Delay Kernel Values RAM 4/11(Kernel 18 Bit Value 10) -> Frame 12 Bit Value 58/1
  Frame 12 Bit Bin Value 4/1 -> Delay Kernel Values RAM 0/5(Frame 12 Bit Bin Value 4)
  Frame 12 Bit Bin Value 53/1 -> Delay Kernel Values RAM 4/6(Frame 12 Bit Bin Value 5)
  Frame 12 Bit Bin Value 11/1 -> Delay Kernel Values RAM 0/12(Frame 12 Bit Bin Value 11)
  Delay Kernel Values RAM 3/6(Kernel 18 Bit Value 5) -> Frame 12 Bit Value 41/1
  Delay Kernel Values RAM 2/5(Kernel 18 Bit Value 4) -> Frame 12 Bit Value 28/1
  Delay Kernel Values RAM 2/11(Kernel 18 Bit Value 10) -> Frame 12 Bit Value 34/1
  Frame 12 Bit Bin Value 59/1 -> Delay Kernel Values RAM 4/12(Frame 12 Bit Bin Value 11)
  Frame 12 Bit Bin Value 0/1 -> Delay Kernel Values RAM 0/1(Frame 12 Bit Bin Value 0)
  Frame 12 Bit Bin Value 38/1 -> Delay Kernel Values RAM 3/3(Frame 12 Bit Bin Value 2)
  Frame 12 Bit Bin Value 16/1 -> Delay Kernel Values RAM 1/5(Frame 12 Bit Bin Value 4)
  Frame 12 Bit Bin Value 18/1 -> Delay Kernel Values RAM 1/7(Frame 12 Bit Bin Value 6)
  Frame 12 Bit Bin Value 27/1 -> Delay Kernel Values RAM 2/4(Frame 12 Bit Bin Value 3)
  Delay Kernel Values RAM 2/1(Kernel 18 Bit Value 0) -> Frame 12 Bit Value 24/1
  Frame 12 Bit Bin Value 22/1 -> Delay Kernel Values RAM 1/11(Frame 12 Bit Bin Value 10)
  Frame 12 Bit Bin Value 34/1 -> Delay Kernel Values RAM 2/11(Frame 12 Bit Bin Value 10)
  Frame 12 Bit Bin Value 3/1 -> Delay Kernel Values RAM 0/4(Frame 12 Bit Bin Value 3)
  Frame 12 Bit Bin Value 58/1 -> Delay Kernel Values RAM 4/11(Frame 12 Bit Bin Value 10)
  Delay Kernel Values RAM 3/3(Kernel 18 Bit Value 2) -> Frame 12 Bit Value 38/1
  Frame 12 Bit Bin Value 39/1 -> Delay Kernel Values RAM 3/4(Frame 12 Bit Bin Value 3)
  Delay Kernel Values RAM 0/6(Kernel 18 Bit Value 5) -> Frame 12 Bit Value 5/1
  Frame 12 Bit Bin Value 49/1 -> Delay Kernel Values RAM 4/2(Frame 12 Bit Bin Value 1)
  Frame 12 Bit Bin Value 8/1 -> Delay Kernel Values RAM 0/9(Frame 12 Bit Bin Value 8)
  Frame 12 Bit Bin Value 35/1 -> Delay Kernel Values RAM 2/12(Frame 12 Bit Bin Value 11)
  Frame 12 Bit Bin Value 14/1 -> Delay Kernel Values RAM 1/3(Frame 12 Bit Bin Value 2)
  Frame 12 Bit Bin Value 44/1 -> Delay Kernel Values RAM 3/9(Frame 12 Bit Bin Value 8)
  Frame 12 Bit Bin Value 56/1 -> Delay Kernel Values RAM 4/9(Frame 12 Bit Bin Value 8)
  Frame 12 Bit Bin Value 36/1 -> Delay Kernel Values RAM 3/1(Frame 12 Bit Bin Value 0)
  Frame 12 Bit Bin Value 29/1 -> Delay Kernel Values RAM 2/6(Frame 12 Bit Bin Value 5)
  Frame 12 Bit Bin Value 7/1 -> Delay Kernel Values RAM 0/8(Frame 12 Bit Bin Value 7)
  Frame 12 Bit Bin Value 31/1 -> Delay Kernel Values RAM 2/8(Frame 12 Bit Bin Value 7)
  Frame 12 Bit Bin Value 45/1 -> Delay Kernel Values RAM 3/10(Frame 12 Bit Bin Value 9)
  Delay Kernel Values RAM 0/10(Kernel 18 Bit Value 9) -> Frame 12 Bit Value 9/1
  Frame 12 Bit Bin Value 40/1 -> Delay Kernel Values RAM 3/5(Frame 12 Bit Bin Value 4)
  Frame 12 Bit Bin Value 23/1 -> Delay Kernel Values RAM 1/12(Frame 12 Bit Bin Value 11)
  Frame 12 Bit Bin Value 46/1 -> Delay Kernel Values RAM 3/11(Frame 12 Bit Bin Value 10)
  Frame 12 Bit Bin Value 5/1 -> Delay Kernel Values RAM 0/6(Frame 12 Bit Bin Value 5)
  Frame 12 Bit Bin Value 10/1 -> Delay Kernel Values RAM 0/11(Frame 12 Bit Bin Value 10)
  Delay Kernel Values RAM 1/4(Kernel 18 Bit Value 3) -> Frame 12 Bit Value 15/1
  Frame 12 Bit Bin Value 32/1 -> Delay Kernel Values RAM 2/9(Frame 12 Bit Bin Value 8)
  Frame 12 Bit Bin Value 55/1 -> Delay Kernel Values RAM 4/8(Frame 12 Bit Bin Value 7)
  Frame 12 Bit Bin Value 1/1 -> Delay Kernel Values RAM 0/2(Frame 12 Bit Bin Value 1)
  Frame 12 Bit Bin Value 30/1 -> Delay Kernel Values RAM 2/7(Frame 12 Bit Bin Value 6)
  Frame 12 Bit Bin Value 24/1 -> Delay Kernel Values RAM 2/1(Frame 12 Bit Bin Value 0)
  Frame 12 Bit Bin Value 47/1 -> Delay Kernel Values RAM 3/12(Frame 12 Bit Bin Value 11)
  Frame 12 Bit Bin Value 54/1 -> Delay Kernel Values RAM 4/7(Frame 12 Bit Bin Value 6)
  Frame 12 Bit Bin Value 41/1 -> Delay Kernel Values RAM 3/6(Frame 12 Bit Bin Value 5)
  Frame 12 Bit Bin Value 6/1 -> Delay Kernel Values RAM 0/7(Frame 12 Bit Bin Value 6)
  Frame 12 Bit Bin Value 48/1 -> Delay Kernel Values RAM 4/1(Frame 12 Bit Bin Value 0)
  Frame 12 Bit Bin Value 33/1 -> Delay Kernel Values RAM 2/10(Frame 12 Bit Bin Value 9)
  Delay Kernel Values RAM 0/2(Kernel 18 Bit Value 1) -> Frame 12 Bit Value 1/1
  Frame 12 Bit Bin Value 25/1 -> Delay Kernel Values RAM 2/2(Frame 12 Bit Bin Value 1)
  Frame 12 Bit Bin Value 15/1 -> Delay Kernel Values RAM 1/4(Frame 12 Bit Bin Value 3)
  Frame 12 Bit Bin Value 20/1 -> Delay Kernel Values RAM 1/9(Frame 12 Bit Bin Value 8)
  Frame 12 Bit Bin Value 51/1 -> Delay Kernel Values RAM 4/4(Frame 12 Bit Bin Value 3)
  Frame 12 Bit Bin Value 19/1 -> Delay Kernel Values RAM 1/8(Frame 12 Bit Bin Value 7)
  Frame 12 Bit Bin Value 43/1 -> Delay Kernel Values RAM 3/8(Frame 12 Bit Bin Value 7)
  Frame 12 Bit Bin Value 9/1 -> Delay Kernel Values RAM 0/10(Frame 12 Bit Bin Value 9)
  Frame 12 Bit Bin Value 52/1 -> Delay Kernel Values RAM 4/5(Frame 12 Bit Bin Value 4)
  Delay Kernel Values RAM 4/6(Kernel 18 Bit Value 5) -> Frame 12 Bit Value 53/1
  Frame 12 Bit Bin Value 17/1 -> Delay Kernel Values RAM 1/6(Frame 12 Bit Bin Value 5)
  Frame 12 Bit Bin Value 13/1 -> Delay Kernel Values RAM 1/2(Frame 12 Bit Bin Value 1)
  Frame 12 Bit Bin Value 28/1 -> Delay Kernel Values RAM 2/5(Frame 12 Bit Bin Value 4)
  Delay Kernel Values RAM 0/11(Kernel 18 Bit Value 10) -> Frame 12 Bit Value 10/1
  Delay Kernel Values RAM 1/2(Kernel 18 Bit Value 1) -> Frame 12 Bit Value 13/1
  Frame 12 Bit Bin Value 12/1 -> Delay Kernel Values RAM 1/1(Frame 12 Bit Bin Value 0)
  Frame 12 Bit Bin Value 42/1 -> Delay Kernel Values RAM 3/7(Frame 12 Bit Bin Value 6)
  Frame 12 Bit Bin Value 50/1 -> Delay Kernel Values RAM 4/3(Frame 12 Bit Bin Value 2)
  Delay Kernel Values RAM 1/10(Kernel 18 Bit Value 9) -> Frame 12 Bit Value 21/1
  Frame 12 Bit Bin Value 57/1 -> Delay Kernel Values RAM 4/10(Frame 12 Bit Bin Value 9)
  Delay Kernel Values RAM 0/1(Kernel 18 Bit Value 0) -> Frame 12 Bit Value 0/1
  Delay Kernel Values RAM 3/1(Kernel 18 Bit Value 0) -> Frame 12 Bit Value 36/1
  Delay Kernel Values RAM 0/4(Kernel 18 Bit Value 3) -> Frame 12 Bit Value 3/1
  Delay Kernel Values RAM 0/3(Kernel 18 Bit Value 2) -> Frame 12 Bit Value 2/1
  Delay Kernel Values RAM 0/5(Kernel 18 Bit Value 4) -> Frame 12 Bit Value 4/1
  Delay Kernel Values RAM 1/1(Kernel 18 Bit Value 0) -> Frame 12 Bit Value 12/1
  Delay Kernel Values RAM 0/12(Kernel 18 Bit Value 11) -> Frame 12 Bit Value 11/1
  Delay Kernel Values RAM 0/9(Kernel 18 Bit Value 8) -> Frame 12 Bit Value 8/1
  Delay Kernel Values RAM 0/8(Kernel 18 Bit Value 7) -> Frame 12 Bit Value 7/1
  Delay Kernel Values RAM 3/2(Kernel 18 Bit Value 1) -> Frame 12 Bit Value 37/1
  Delay Kernel Values RAM 1/11(Kernel 18 Bit Value 10) -> Frame 12 Bit Value 22/1
  Delay Kernel Values RAM 3/5(Kernel 18 Bit Value 4) -> Frame 12 Bit Value 40/1
  Delay Kernel Values RAM 3/7(Kernel 18 Bit Value 6) -> Frame 12 Bit Value 42/1
  Delay Kernel Values RAM 3/4(Kernel 18 Bit Value 3) -> Frame 12 Bit Value 39/1
  Delay Kernel Values RAM 3/10(Kernel 18 Bit Value 9) -> Frame 12 Bit Value 45/1
  Delay Kernel Values RAM 3/8(Kernel 18 Bit Value 7) -> Frame 12 Bit Value 43/1
  Delay Kernel Values RAM 4/1(Kernel 18 Bit Value 0) -> Frame 12 Bit Value 48/1
  Delay Kernel Values RAM 3/9(Kernel 18 Bit Value 8) -> Frame 12 Bit Value 44/1
  Delay Kernel Values RAM 3/11(Kernel 18 Bit Value 10) -> Frame 12 Bit Value 46/1
  Delay Kernel Values RAM 1/5(Kernel 18 Bit Value 4) -> Frame 12 Bit Value 16/1
  Delay Kernel Values RAM 3/12(Kernel 18 Bit Value 11) -> Frame 12 Bit Value 47/1
  Delay Kernel Values RAM 1/3(Kernel 18 Bit Value 2) -> Frame 12 Bit Value 14/1
  Delay Kernel Values RAM 1/9(Kernel 18 Bit Value 8) -> Frame 12 Bit Value 20/1
  Delay Kernel Values RAM 1/7(Kernel 18 Bit Value 6) -> Frame 12 Bit Value 18/1
  Delay Kernel Values RAM 1/8(Kernel 18 Bit Value 7) -> Frame 12 Bit Value 19/1
  Delay Kernel Values RAM 4/2(Kernel 18 Bit Value 1) -> Frame 12 Bit Value 49/1
  Delay Kernel Values RAM 1/6(Kernel 18 Bit Value 5) -> Frame 12 Bit Value 17/1
  Delay Kernel Values RAM 4/7(Kernel 18 Bit Value 6) -> Frame 12 Bit Value 54/1
  Delay Kernel Values RAM 1/12(Kernel 18 Bit Value 11) -> Frame 12 Bit Value 23/1
  Delay Kernel Values RAM 4/3(Kernel 18 Bit Value 2) -> Frame 12 Bit Value 50/1
  Delay Kernel Values RAM 4/4(Kernel 18 Bit Value 3) -> Frame 12 Bit Value 51/1
  Delay Kernel Values RAM 4/5(Kernel 18 Bit Value 4) -> Frame 12 Bit Value 52/1
  Delay Kernel Values RAM 4/8(Kernel 18 Bit Value 7) -> Frame 12 Bit Value 55/1
  Delay Kernel Values RAM 2/12(Kernel 18 Bit Value 11) -> Frame 12 Bit Value 35/1
  Delay Kernel Values RAM 4/9(Kernel 18 Bit Value 8) -> Frame 12 Bit Value 56/1
  Delay Kernel Values RAM 2/2(Kernel 18 Bit Value 1) -> Frame 12 Bit Value 25/1
  Delay Kernel Values RAM 4/10(Kernel 18 Bit Value 9) -> Frame 12 Bit Value 57/1
  Delay Kernel Values RAM 4/12(Kernel 18 Bit Value 11) -> Frame 12 Bit Value 59/1
  Delay Kernel Values RAM 2/6(Kernel 18 Bit Value 5) -> Frame 12 Bit Value 29/1
  Delay Kernel Values RAM 2/8(Kernel 18 Bit Value 7) -> Frame 12 Bit Value 31/1
  Delay Kernel Values RAM 2/3(Kernel 18 Bit Value 2) -> Frame 12 Bit Value 26/1
  Delay Kernel Values RAM 2/7(Kernel 18 Bit Value 6) -> Frame 12 Bit Value 30/1
  Delay Kernel Values RAM 2/10(Kernel 18 Bit Value 9) -> Frame 12 Bit Value 33/1
  Delay Kernel Values RAM 2/9(Kernel 18 Bit Value 8) -> Frame 12 Bit Value 32/1
